simulink model "system_simulation"  (R2021a)
settings: Solver=VariableStepAuto  StartTime=0.0  StopTime=1.016  RelTol=1e-3
settings Model: Creator=Musthafa  LastModifiedBy=Musthafa

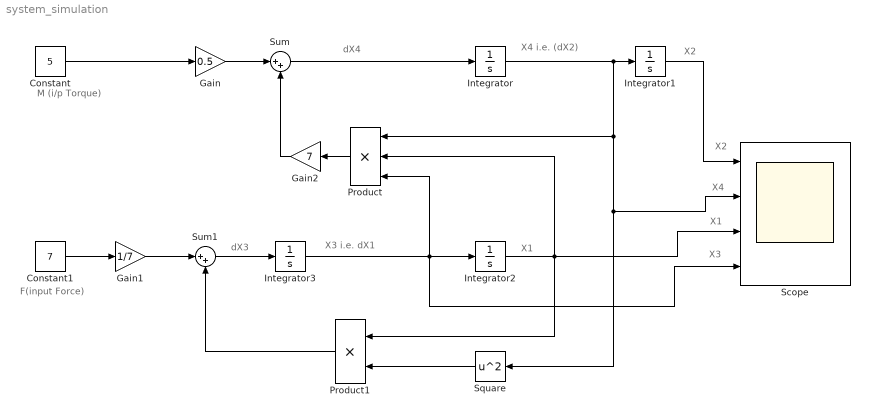
== system system_simulation ==
  note: dX3
  note: X3 i.e. dX1
  note: X1
  note: X2
  note: X4 i.e. (dX2)
  note: dX4
  note: X3
  note: X1
  note: X4
  note: X2
  note: F(input Force)
  note: M (i/p Torque)
  Constant : Constant  Value=5
  Constant1 : Constant  Value=7
  Gain : Gain  Gain=0.5
  Gain1 : Gain  Gain=1/7
  Gain2 : Gain  Gain=7
  Integrator{,1..3} (4 alike) : Integrator
  Product : Product  Inputs=3
  Product1 : Product
  Scope : Scope  NumInputPorts=4
  Square : Math  Operator=square  SaturateOnIntegerOverflow=on
  Sum : Sum  Inputs=|++
  Sum1 : Sum  Inputs=|++
  wires:
  Constant/1 -> Gain/1
  Gain/1 -> Sum/1
  Sum/1 -> Integrator/1
  Integrator/1 -> Product/1, Scope/2, Square/1, Integrator1/1
  Integrator1/1 -> Scope/1
  Gain2/1 -> Sum/2
  Product/1 -> Gain2/1
  Square/1 -> Product1/2
  Constant1/1 -> Gain1/1
  Gain1/1 -> Sum1/1
  Product1/1 -> Sum1/2
  Sum1/1 -> Integrator3/1
  Integrator3/1 -> Integrator2/1, Scope/4, Product/3
  Integrator2/1 -> Product1/1, Product/2, Scope/3
